simulink model "Fig220"  (R2014a)
settings: Solver=ode3  StartTime=0.0  StopTime=5.24288  FixedStep=2e-5  RelTol=1e-5
undefined symbols (not defined in the file): gcbh, rcfiltgaincompat
libraries: commrandsrc2 x1, commfilt2 x1
settings Model: Creator=Dennis Silage  LastModifiedBy=Silage
settings DataIOCC: SignalLoggingSaveFormat=ModelDataLogs
settings OptimizationCC: ExpressionDepthLimit=2147483647  InitFltsAndDblsToZero=on
settings DebuggingCC: UnderspecifiedInitializationDetection=Classic  SolverPrmCheckMsg=none  FcnCallInpInsideContextMsg=UseLocalSettings  StateNameClashWarn=warning
settings GRTTargetCC: CombineOutputUpdateFcns=off  GRTInterface=on

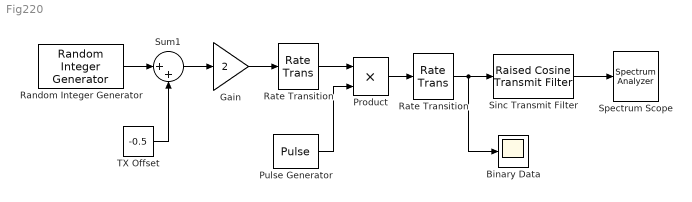
== system Fig220 ==
  " Rate Transition" : RateTransition  OutPortSampleTime=1e-3
  Binary Data : Scope
      settings: YMin=-1.5  YMax=1.5
  Gain : Gain  Gain=2
  Product : Product  RndMeth=Zero
  Pulse Generator : DiscretePulseGenerator  PulseType=Time based  Period=1e-3  PulseWidth=2
  Random Integer Generator : commrandsrc2/Random Integer Generator  mul=2  seed=randseed  Ts=1e-3  frameBased=off  sampPerFrame=50  orient=off  outDataType=double
  Rate Transition : RateTransition  OutPortSampleTime=2e-5
  Sinc Transmit Filter : commfilt2/Raised Cosine Transmit Filter  filtType=Normal  filtSpan=2*(4)  currentFiltSpan=2*(4)  D=4  R=0  sampMode=Mute  saveAsFlag=0  N=50  framing=Maintain input frame size  InputProcessing=Inherited (this choice will be removed - see release notes)  checkGain=User-specified  filterGain=(5)*rcfiltgaincompat(gcbh)  checkCoeff=off  variableName=rcTxFilt  launchFVT=off  roundingMode=Floor  overflowMode=off
  Spectrum Scope : SpectrumAnalyzer
  Sum1 : Sum  Inputs=|++
  TX Offset : Constant  Value=-0.5
  wires:
  Sum1/1 -> Gain/1
  TX Offset/1 -> Sum1/2
  Random Integer Generator/1 -> Sum1/1
  Gain/1 -> Rate Transition/1
  Rate Transition/1 -> Product/1
  Pulse Generator/1 -> Product/2
  Sinc Transmit Filter/1 -> Spectrum Scope/1
  " Rate Transition"/1 -> Sinc Transmit Filter/1, Binary Data/1
  Product/1 -> " Rate Transition"/1
